simulink model "Circuits"  (R2025b)
settings: Solver=VariableStepAuto  StartTime=0.0  StopTime=10.0  RelTol=1e-3
undefined symbols (not defined in the file): hw
libraries: nvidiaAVlib x4, raspberrypiAVlib x1

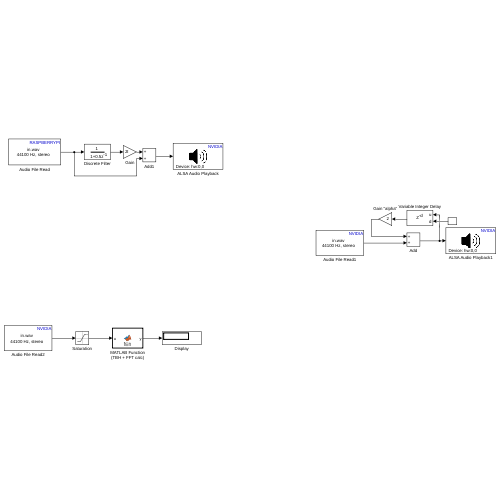
[thumbnail: Simulink's stored preview of the top-level diagram]
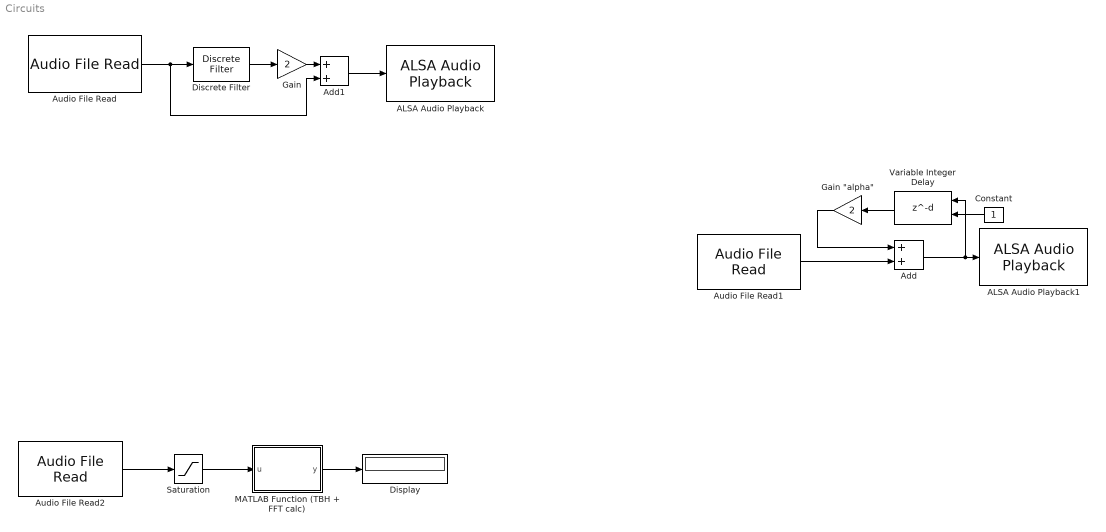
== system Circuits ==
  ALSA Audio Playback : nvidiaAVlib/ALSA Audio Playback  deviceStr=hw:0,0  sampleRateEnum=44100  queueDuration=0.5  blockPlatform=LINUX
  ALSA Audio Playback1 : nvidiaAVlib/ALSA Audio Playback  deviceStr=hw:0,0  sampleRateEnum=44100  queueDuration=0.5  blockPlatform=LINUX
  Add : Sum
  Add1 : Sum
  Audio File Read : raspberrypiAVlib/Audio File Read  FileName=/MATLAB Drive/Projects/untitled/in.wav  PlayCount=Inf  OutputEOFIndicator=off  SamplesPerFrame=4410
  Audio File Read1 : nvidiaAVlib/Audio File Read  FileName=in.wav  PlayCount=Inf  OutputEOFIndicator=off  SamplesPerFrame=4410
  Audio File Read2 : nvidiaAVlib/Audio File Read  FileName=in.wav  PlayCount=Inf  OutputEOFIndicator=off  SamplesPerFrame=4410
  Constant : Constant
  Discrete Filter : DiscreteFilter
  Display : Display
  Gain : Gain  Gain=2
  "Gain \"alpha\"" : Gain  Gain=2
  MATLAB Function (TBH + FFT calc) : MATLAB Function  TreatAsAtomicUnit=on
  Saturation : Saturate  UpperLimit=15  LowerLimit=-15
  Variable Integer Delay : Delay  DelayLengthSource=Input port
      settings: InputPortMap=u0,p1
  wires:
  Audio File Read1/1 -> Add/2
  Variable Integer Delay/1 -> "Gain \"alpha\""/1
  "Gain \"alpha\""/1 -> Add/1
  Add/1 -> Variable Integer Delay/1, ALSA Audio Playback1/1
  MATLAB Function (TBH + FFT calc)/1(y) -> Display/1
  Saturation/1 -> MATLAB Function (TBH + FFT calc)/1(u)
  Audio File Read2/1 -> Saturation/1
  Discrete Filter/1 -> Gain/1
  Audio File Read/1 -> Add1/2, Discrete Filter/1
  Gain/1 -> Add1/1
  Add1/1 -> ALSA Audio Playback/1
  Constant/1 -> Variable Integer Delay/2

== matlab function Circuits/MATLAB Function (TBH + FFT calc) ==
  data: u input; y output
function y = fcn(u)

y = u;
